simulink model "actuator"  (R2021a)
settings: Solver=FixedStepAuto  StartTime=start_time  StopTime=stop_time  FixedStep=min_step  RelTol=1e-3
values from neighbouring files (symbols this model uses):
  alpha = 5000    [controlprj.m]
  amp = 2000    [controlprj.m]
  c = 0    [controlprj.m]
  delta_t = 0.001    [controlprj.m]
  g = 9.80665    [controlprj.m]
  initial_disp = 0.01    [controlprj.m]
  initial_velocity = 0.1    [controlprj.m]
  k = 29127    [controlprj.m]
  m = 5873    [controlprj.m]
  switchF = 1    [controlprj.m]
  target_t = 30    [controlprj.m]
libraries: simulink x1, fuzblock x1
settings Model: Creator=mehrab  LastModifiedBy=mehrab
settings SolverCC: AlgebraicLoopSolver=TrustRegion
settings DataIOCC: ReturnWorkspaceOutputs=off
settings DebuggingCC: SFMachineParentedDataDiag=warning  UnderSpecifiedDimensionMsg=warning  ArithmeticOperatorsInVariantConditions=warning
settings SFSimCC: SimUseLocalCustomCode=off  CustomCodeUndefinedFunction=UseInterfaceOnly
settings RTWCC: RTWUseLocalCustomCode=off

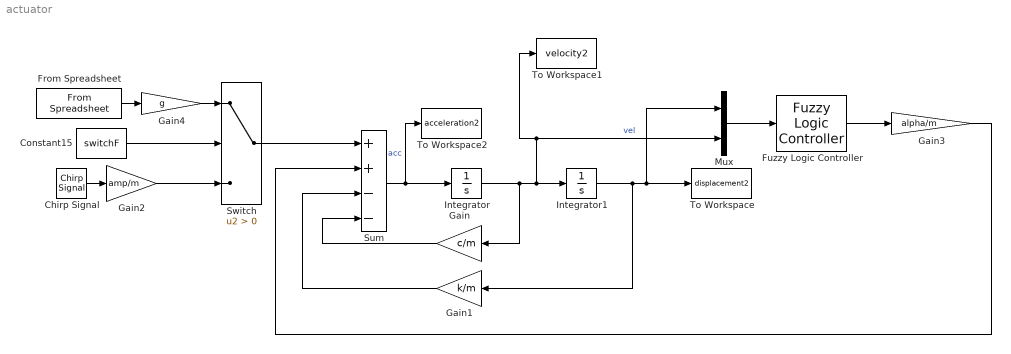
== system actuator ==
  Chirp Signal : simulink/Sources/Chirp Signal  f1=initial_freq  T=target_t  f2=freq_target
  Constant15 : Constant  Value=switchF
  From Spreadsheet : FromSpreadsheet  FileName=elcentro.xlsx
  Fuzzy Logic Controller : fuzblock/Fuzzy Logic  Controller  FIS='actuatorfuzzy'  OutputSampleNumber=101  DataType=double  FuzzifiedInputs=off  RuleFiringStrengths=off  RuleOutputs=off  AggregatedOutputs=off  SimulateUsing=Interpreted execution  OutOfRangeInputValueMessage=warning  NoRuleFiredMessage=warning  EmptyOutputFuzzySetMessage=warning
  Gain : Gain  Gain=c/m
  Gain1 : Gain  Gain=k/m
  Gain2 : Gain  Gain=amp/m
  Gain3 : Gain  Gain=alpha/m
  Gain4 : Gain  Gain=g
  Integrator : Integrator  InitialCondition=initial_velocity
  Integrator1 : Integrator  InitialCondition=initial_disp
  Mux : Mux  Inputs=2
  Sum : Sum  Inputs=++--
  Switch : Switch  Criteria=u2 > Threshold
  To Workspace : ToWorkspace  VariableName=displacement2  SampleTime=delta_t
  To Workspace1 : ToWorkspace  VariableName=velocity2  SampleTime=delta_t
  To Workspace2 : ToWorkspace  VariableName=acceleration2  SampleTime=delta_t
  wires:
  Chirp Signal/1 -> Gain2/1
  Sum/1 -> To Workspace2/1, Integrator/1  "acc"
  Integrator/1 -> To Workspace1/1, Mux/2, Integrator1/1, Gain/1  "vel"
  Gain/1 -> Sum/4
  Gain1/1 -> Sum/3
  Mux/1 -> Fuzzy Logic Controller/1
  Integrator1/1 -> Mux/1, To Workspace/1, Gain1/1
  Switch/1 -> Sum/1
  Gain2/1 -> Switch/3
  Constant15/1 -> Switch/2
  Gain4/1 -> Switch/1
  From Spreadsheet/1 -> Gain4/1
  Fuzzy Logic Controller/1 -> Gain3/1
  Gain3/1 -> Sum/2
